simulink model "digital_control_4_2_3"  (R2021b)
settings: Solver=VariableStepAuto  StartTime=0.0  StopTime=10.0  RelTol=1e-3
values from neighbouring files (symbols this model uses):
  d_den = cell2mat(d_den)    [in_lab.m]
  d_num = cell2mat(d_num)    [in_lab.m]
  f1 = F(1)    [in_lab.m]
  T = 0.05    [in_lab.m]
  u_bar = sqrt(g*x_bar(1)^2)    [in_lab.m]    (also in prelab.m)
  x_bar = [0.5; 0.0]    [in_lab.m]    (also in prelab.m)
settings Model: Creator=pranshumalik14  LastModifiedBy=varunsampat
settings SolverCC: AlgebraicLoopSolver=TrustRegion
settings DataIOCC: ReturnWorkspaceOutputs=off
settings DebuggingCC: SFMachineParentedDataDiag=warning  ArithmeticOperatorsInVariantConditions=warning
settings SFSimCC: CustomCodeUndefinedFunction=UseInterfaceOnly

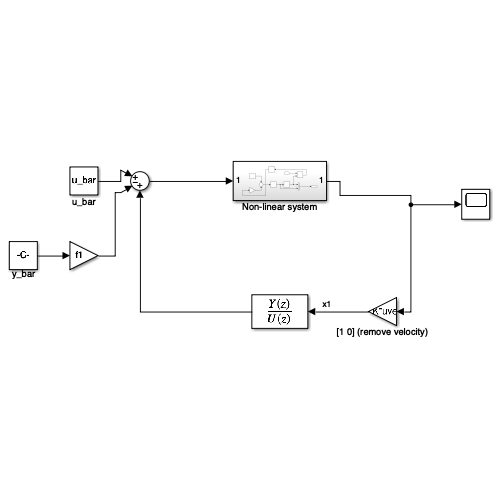
[thumbnail: Simulink's stored preview of the top-level diagram]
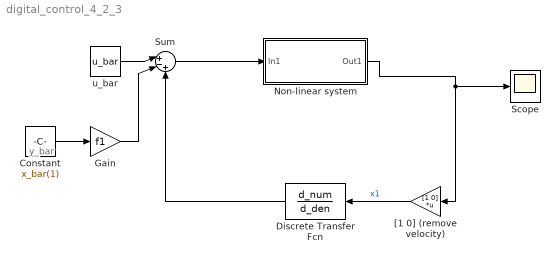
== system digital_control_4_2_3 ==
  note: y_bar
  Constant : Constant  Value=x_bar(1)
  Discrete Transfer Fcn : DiscreteTransferFcn  Numerator=d_num  Denominator=d_den  SampleTime=T
  Gain : Gain  Gain=f1
  Non-linear system : Subsystem
  Scope : Scope
  Sum : Sum  Inputs=|+-+
  "[1 0] (remove velocity)" : Gain  Gain=[1 0]  Multiplication=Matrix(K*u) (u vector)
  u_bar : Constant  Value=u_bar
  wires:
  Non-linear system/1(Out1) -> "[1 0] (remove velocity)"/1, Scope/1
  u_bar/1 -> Sum/1
  Sum/1 -> Non-linear system/1(In1)
  Constant/1 -> Gain/1
  Gain/1 -> Sum/2
  Discrete Transfer Fcn/1 -> Sum/3
  "[1 0] (remove velocity)"/1 -> Discrete Transfer Fcn/1  "x1"

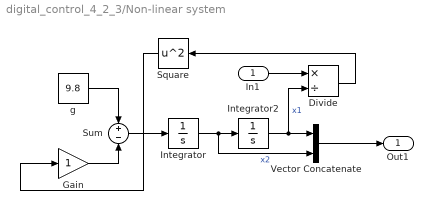
== system digital_control_4_2_3/Non-linear system ==
  In1 : Inport
  Divide : Product  Inputs=*/
  Gain : Gain
  Integrator : Integrator  InitialCondition=0.5
  Integrator2 : Integrator  InitialCondition=16
  Square : Math  Operator=square  SignedPower=on  SaturateOnIntegerOverflow=on
  Sum : Sum  Inputs=+-
  Vector Concatenate : Concatenate
  g : Constant  Value=9.8
  Out1 : Outport  VectorParamsAs1DForOutWhenUnconnected=off
  wires:
  Integrator2/1 -> Vector Concatenate/1, Divide/2  "x1"
  Integrator/1 -> Vector Concatenate/2, Integrator2/1  "x2"
  Vector Concatenate/1 -> Out1/1
  Divide/1 -> Square/1
  Square/1 -> Gain/1
  In1/1 -> Divide/1
  Gain/1 -> Sum/2
  g/1 -> Sum/1
  Sum/1 -> Integrator/1
